simulink model "a_201532004_8_1"  (Simulink 7.7)
settings: Solver=ode45  StartTime=0.0  StopTime=10.0  RelTol=1e-3
settings Model: Creator=Administrator  LastModifiedBy=Administrator

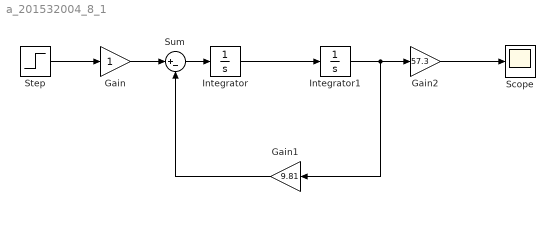
== system a_201532004_8_1 ==
  Gain : Gain
  Gain1 : Gain  Gain=9.81
  Gain2 : Gain  Gain=57.3
  Integrator : Integrator
  Integrator1 : Integrator
  Scope : Scope
  Step : Step  SampleTime=0
  Sum : Sum  Inputs=|+-
  wires:
  Step/1 -> Gain/1
  Gain/1 -> Sum/1
  Integrator/1 -> Integrator1/1
  Integrator1/1 -> Gain2/1, Gain1/1
  Sum/1 -> Integrator/1
  Gain1/1 -> Sum/2
  Gain2/1 -> Scope/1
